simulink model "sim_main_esb_7"  (R2018b)
settings: Solver=VariableStepAuto  StartTime=0.0  StopTime=10.0  RelTol=1e-3
values from neighbouring files (symbols this model uses):
  A = 0.914    [KALMAN.m]    (also in main_cntl.m = eval(A_eq); main_sys.m = double(A_lin); main_sys_klm.m = double(A_lin); main_tf_0.m = A)
  B_1 = B(:,1)    [main_tf_6.m]
  C = 0.344    [KALMAN.m]    (also in main_sys.m = double( subs( C) ); main_sys_klm.m = double( subs( C) ); main_tf_0.m = [ 0 , 0  , Ks , ds , -Ks , -ds, 0 ]; main_tf_1.m = C_mes)
  D = zeros(7,2)    [main_sys.m]    (also in main_sys_klm.m = zeros(2,2); main_tf_0.m = [ 0 , 0 ]; main_tf_1.m = zeros(1,1); main_tf_10.m = zeros(2,2))
  K = P*C'/(C*P*C' + R)    [KALMAN.m]    (also in main_tf_9.m = lqi(sys_lq,Q,R))
undefined symbols (not defined in the file or in its folder): kalmf
settings Model: Creator=eshojaei  LastModifiedBy=eshojaei

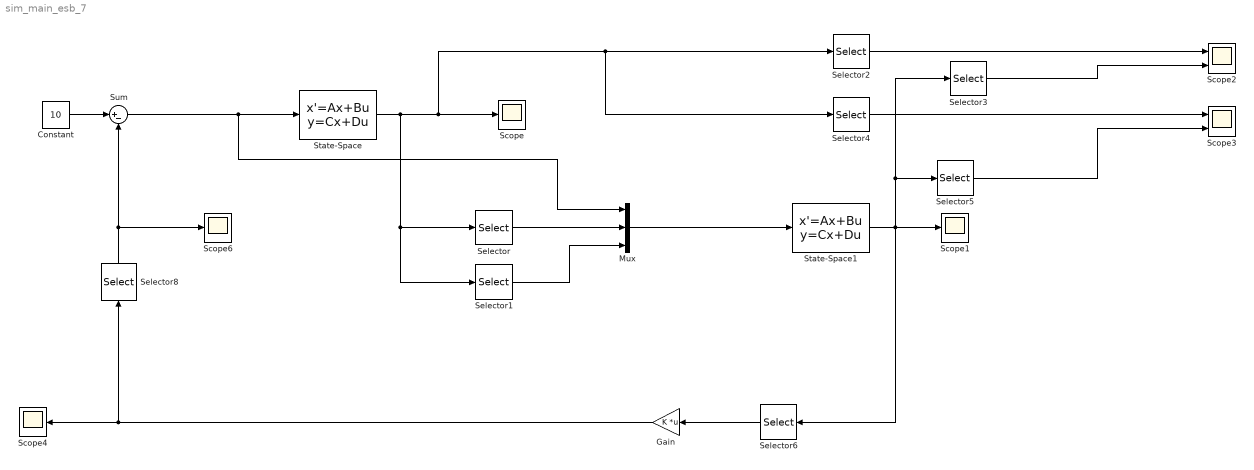
== system sim_main_esb_7 ==
  Constant : Constant  Value=10
  Gain : Gain  Gain=K  Multiplication=Matrix(K*u)
  Mux : Mux  Inputs=3
  Scope{,1,4,6} (4 alike) : Scope
  Scope2 : Scope  NumInputPorts=2
  Scope3 : Scope  NumInputPorts=2
  Selector : Selector  InputPortWidth=2  IndexOptions=Index vector (dialog)  Indices=[1]  OutputSizes=1
  Selector1 : Selector  InputPortWidth=2  IndexOptions=Index vector (dialog)  Indices=[2]  OutputSizes=1
  Selector2 : Selector  InputPortWidth=2  IndexOptions=Index vector (dialog)  Indices=[1]  OutputSizes=1
  Selector3 : Selector  InputPortWidth=9  IndexOptions=Index vector (dialog)  Indices=[1]  OutputSizes=1
  Selector4 : Selector  InputPortWidth=2  IndexOptions=Index vector (dialog)  Indices=[2]  OutputSizes=1
  Selector5 : Selector  InputPortWidth=9  IndexOptions=Index vector (dialog)  Indices=[2]  OutputSizes=1
  Selector6 : Selector  InputPortWidth=9  IndexOptions=Index vector (dialog)  Indices=[3:9]  OutputSizes=1
  Selector8 : Selector  InputPortWidth=2  IndexOptions=Index vector (dialog)  Indices=[1]  OutputSizes=1
  State-Space : StateSpace  A=A  B=B_1  C=C  D=D  InitialCondition=0
  State-Space1 : StateSpace  A=kalmf.A  B=kalmf.B  C=kalmf.C  D=kalmf.D  InitialCondition=0
  Sum : Sum  Inputs=|+-
  wires:
  Sum/1 -> Mux/1, State-Space/1
  State-Space/1 -> Selector1/1, Selector/1, Selector4/1, Selector2/1, Scope/1
  Mux/1 -> State-Space1/1
  State-Space1/1 -> Selector6/1, Selector5/1, Selector3/1, Scope1/1
  Selector/1 -> Mux/2
  Selector1/1 -> Mux/3
  Selector2/1 -> Scope2/1
  Selector3/1 -> Scope2/2
  Selector4/1 -> Scope3/1
  Selector5/1 -> Scope3/2
  Selector6/1 -> Gain/1
  Gain/1 -> Selector8/1, Scope4/1
  Constant/1 -> Sum/1
  Selector8/1 -> Scope6/1, Sum/2
